simulink model "winter_simulink"  (R2022a)
settings: Solver=FixedStepAuto  StartTime=0  StopTime=simulation.stop_time  FixedStep=simulation.time_step  RelTol=1e-3
values from neighbouring files (symbols this model uses):
  I_eq = param{1}    [main_IMM.m]    (also in parameters_old.m = rotor.I + generator.I/gearbox.ratio^2)
  lambda_vector = linspace(lambda_range(1), lambda_range(2), lambda_item)    [parameters_old.m]
  omega_rated = rated_values(2)    [parameters_old.m]
  pitch_range = deg2rad([-15 90])    [parameters_old.m]
  pitch_vector = linspace(pitch_range(1), pitch_range(2), pitch_item)    [parameters_old.m]
  rho = param{2}    [main_IMM.m]    (also in parameters_old.m = 1.225)
undefined symbols (not defined in the file or in its folder): blade, Gc, gearbox, generator, lookup_cP, omega_r, Riq, rotor, wind, Yiq
settings Model: Creator=Niccolò  LastModifiedBy=Niccolò

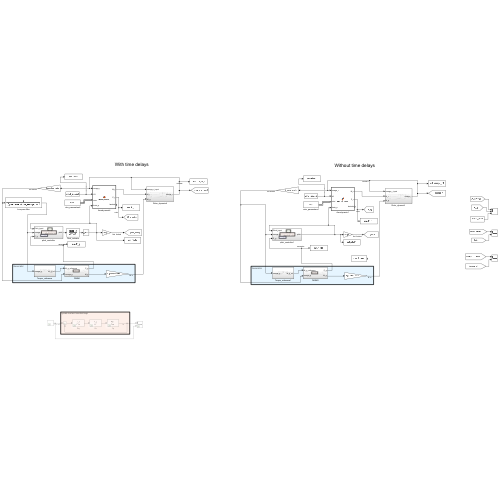
[thumbnail: Simulink's stored preview of the top-level diagram]
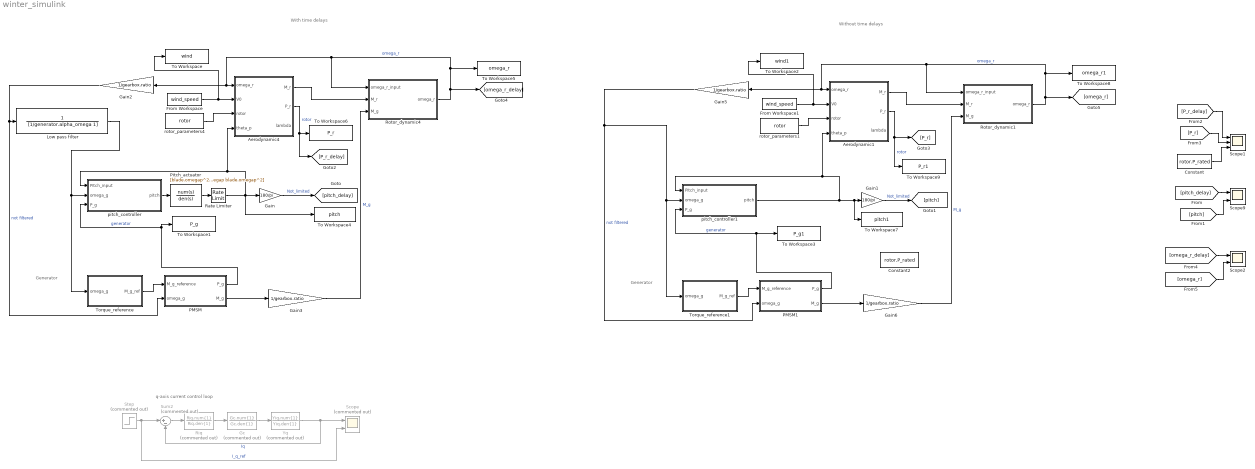
== system winter_simulink ==
  note: Generator
  note: With time delays
  note: q-axis current control loop
  note: Generator
  note: Without time delays
  Aerodynamic1 : MATLAB Function  TreatAsAtomicUnit=on
  Aerodynamic4 : MATLAB Function  TreatAsAtomicUnit=on
  Constant : Constant  Value=rotor.P_rated
  Constant2 : Constant  Value=rotor.P_rated
  From Workspace : FromWorkspace  VariableName=wind_speed  SampleTime=1/wind.sample_f
  From Workspace1 : FromWorkspace  VariableName=wind_speed  SampleTime=1/wind.sample_f
  Gain : Gain  Gain=180/pi
  Gain1 : Gain  Gain=180/pi
  Gain{2..3,5..6} (4 alike) : Gain  Gain=1/gearbox.ratio
  Gc : TransferFcn  Commented=on  Numerator=Gc.num{1}  Denominator=Gc.den{1}
  Low pass filter : TransferFcn  Denominator=[1/generator.alpha_omega 1]
  PMSM : Subsystem
  PMSM1 : Subsystem
  Pitch_actuator : TransferFcn  Numerator=[blade.omegap^2]  Denominator=[1 2*blade.zetap*blade.omegap blade.omegap^2]
  Rate Limiter : RateLimiter  RisingSlewLimit=blade.pitch_rate  FallingSlewLimit=-blade.pitch_rate  SampleTimeMode=inherited
  Riq : TransferFcn  Commented=on  Numerator=Riq.num{1}  Denominator=Riq.den{1}
  Rotor_dynamic1 : Subsystem
  Rotor_dynamic4 : Subsystem
  Scope : Scope  Commented=on  NumInputPorts=2
  Scope1 : Scope  NumInputPorts=3
  Scope2 : Scope  NumInputPorts=2
  Scope9 : Scope  NumInputPorts=2
  Step : Step  Commented=on  SampleTime=0
  Sum2 : Sum  Commented=on  Inputs=|+-
  To Workspace : ToWorkspace  VariableName=wind  SaveFormat=Timeseries  SampleTime=-1
  To Workspace1 : ToWorkspace  VariableName=P_g  SaveFormat=Timeseries  SampleTime=-1
  To Workspace2 : ToWorkspace  VariableName=wind1  SaveFormat=Timeseries  SampleTime=-1
  To Workspace3 : ToWorkspace  VariableName=P_g1  SaveFormat=Timeseries  SampleTime=-1
  To Workspace4 : ToWorkspace  VariableName=pitch  SaveFormat=Timeseries  SampleTime=-1
  To Workspace5 : ToWorkspace  VariableName=omega_r  SaveFormat=Timeseries  SampleTime=-1
  To Workspace6 : ToWorkspace  VariableName=P_r  SaveFormat=Timeseries  SampleTime=-1
  To Workspace7 : ToWorkspace  VariableName=pitch1  SaveFormat=Timeseries  SampleTime=-1
  To Workspace8 : ToWorkspace  VariableName=omega_r1  SaveFormat=Timeseries  SampleTime=-1
  To Workspace9 : ToWorkspace  VariableName=P_r1  SaveFormat=Timeseries  SampleTime=-1
  Torque_reference : Subsystem
  Torque_reference1 : Subsystem
  Yq : TransferFcn  Commented=on  Numerator=Yiq.num{1}  Denominator=Yiq.den{1}
  pitch_controller : Subsystem
  pitch_controller1 : Subsystem
  rotor_parameters1 : Constant  Value=rotor  OutDataTypeStr=Bus: rotor_bus
  rotor_parameters4 : Constant  Value=rotor  OutDataTypeStr=Bus: rotor_bus
  wires:
  Aerodynamic4/1(M_r) -> Rotor_dynamic4/2(M_r)
  From Workspace/1 -> To Workspace/1, Aerodynamic4/2(V0)
  rotor_parameters4/1 -> Aerodynamic4/3(rotor)
  Gain2/1 -> PMSM/2(omega_g), Low pass filter/1  "not filtered"
  Rotor_dynamic4/1(omega_r) -> [omega_r_delay], Rotor_dynamic4/1(omega_r_input), Gain2/1, Aerodynamic4/1(omega_r), To Workspace5/1  "omega_r"
  Aerodynamic4/2(P_r) -> [P_r_delay], To Workspace6/1  "rotor"
  Gain/1 -> [pitch_delay]  "Not_limited"
  PMSM/1(P_g) -> To Workspace1/1, pitch_controller/3(P_g)  "generator"
  Torque_reference/1(M_g_ref) -> PMSM/1(M_g_reference)
  pitch_controller/1(pitch) -> Pitch_actuator/1
  PMSM/2(M_g) -> Gain3/1
  Gain3/1 -> Rotor_dynamic4/3(M_g)  "M_g"
  Step/1 -> Scope/2, Sum2/1  "I_q_ref"
  Gc/1 -> Yq/1
  Riq/1 -> Gc/1
  Yq/1 -> Scope/1, Sum2/2  "Iq"
  Sum2/1 -> Riq/1
  Low pass filter/1 -> Torque_reference/1(omega_g), pitch_controller/2(omega_g)
  Pitch_actuator/1 -> Rate Limiter/1
  Rate Limiter/1 -> Aerodynamic4/4(theta_p), pitch_controller/1(Pitch_input), Gain/1, To Workspace4/1
  pitch_controller1/1(pitch) -> To Workspace7/1, Gain1/1, Aerodynamic1/4(theta_p), pitch_controller1/1(Pitch_input)
  PMSM1/2(M_g) -> Gain6/1
  PMSM1/1(P_g) -> pitch_controller1/3(P_g), To Workspace3/1  "generator"
  Gain6/1 -> Rotor_dynamic1/3(M_g)  "M_g"
  Torque_reference1/1(M_g_ref) -> PMSM1/1(M_g_reference)
  rotor_parameters1/1 -> Aerodynamic1/3(rotor)
  Gain1/1 -> [pitch]  "Not_limited"
  Gain5/1 -> Torque_reference1/1(omega_g), pitch_controller1/2(omega_g), PMSM1/2(omega_g)  "not filtered"
  Aerodynamic1/2(P_r) -> [P_r], To Workspace9/1  "rotor"
  Rotor_dynamic1/1(omega_r) -> [omega_r], Rotor_dynamic1/1(omega_r_input), Gain5/1, Aerodynamic1/1(omega_r), To Workspace8/1  "omega_r"
  From Workspace1/1 -> To Workspace2/1, Aerodynamic1/2(V0)
  Aerodynamic1/1(M_r) -> Rotor_dynamic1/2(M_r)
  [pitch_delay] -> Scope9/1
  [pitch] -> Scope9/2
  [P_r_delay] -> Scope1/1
  [P_r] -> Scope1/2
  Constant/1 -> Scope1/3
  [omega_r_delay] -> Scope2/1
  [omega_r] -> Scope2/2

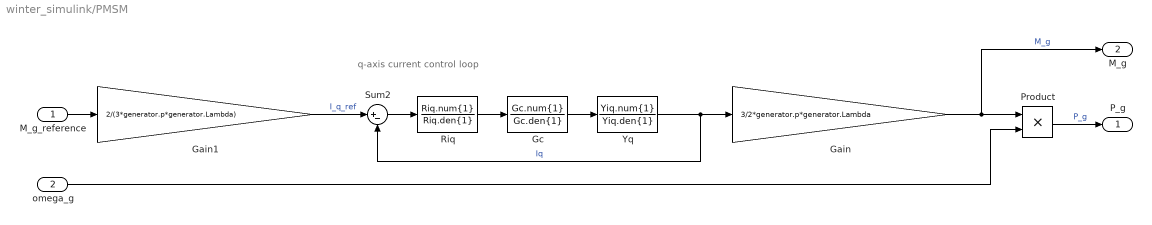
== system winter_simulink/PMSM ==
  note: q-axis current control loop
  M_g_reference : Inport
  omega_g : Inport  Port=2
  Gain : Gain  Gain=3/2*generator.p*generator.Lambda
  Gain1 : Gain  Gain=2/(3*generator.p*generator.Lambda)
  Gc : TransferFcn  Numerator=Gc.num{1}  Denominator=Gc.den{1}
  Product : Product
  Riq : TransferFcn  Numerator=Riq.num{1}  Denominator=Riq.den{1}
  Sum2 : Sum  Inputs=|+-
  Yq : TransferFcn  Numerator=Yiq.num{1}  Denominator=Yiq.den{1}
  P_g : Outport
  M_g : Outport  Port=2
  wires:
  Gc/1 -> Yq/1
  M_g_reference/1 -> Gain1/1
  Gain/1 -> M_g/1, Product/1  "M_g"
  Riq/1 -> Gc/1
  Sum2/1 -> Riq/1
  Yq/1 -> Gain/1, Sum2/2  "Iq"
  Product/1 -> P_g/1  "P_g"
  omega_g/1 -> Product/2
  Gain1/1 -> Sum2/1  "I_q_ref"

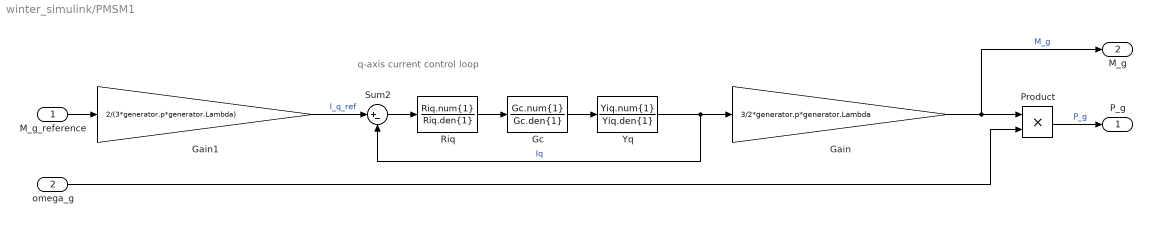
== system winter_simulink/PMSM1 ==
  note: q-axis current control loop
  M_g_reference : Inport
  omega_g : Inport  Port=2
  Gain : Gain  Gain=3/2*generator.p*generator.Lambda
  Gain1 : Gain  Gain=2/(3*generator.p*generator.Lambda)
  Gc : TransferFcn  Numerator=Gc.num{1}  Denominator=Gc.den{1}
  Product : Product
  Riq : TransferFcn  Numerator=Riq.num{1}  Denominator=Riq.den{1}
  Sum2 : Sum  Inputs=|+-
  Yq : TransferFcn  Numerator=Yiq.num{1}  Denominator=Yiq.den{1}
  P_g : Outport
  M_g : Outport  Port=2
  wires:
  Gc/1 -> Yq/1
  M_g_reference/1 -> Gain1/1
  Gain/1 -> M_g/1, Product/1  "M_g"
  Riq/1 -> Gc/1
  Sum2/1 -> Riq/1
  Yq/1 -> Gain/1, Sum2/2  "Iq"
  Product/1 -> P_g/1  "P_g"
  omega_g/1 -> Product/2
  Gain1/1 -> Sum2/1  "I_q_ref"

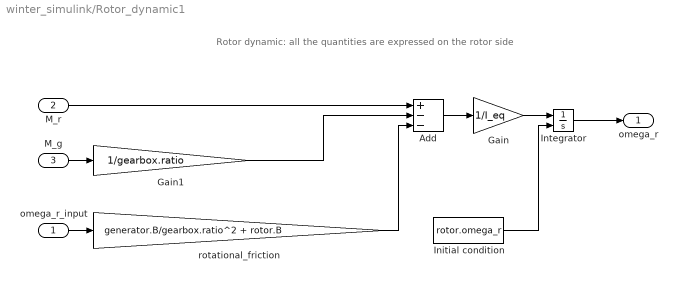
== system winter_simulink/Rotor_dynamic1 ==
  note: Rotor dynamic: all the quantities are expressed on the rotor side
  omega_r_input : Inport
  M_r : Inport  Port=2
  M_g : Inport  Port=3
  Add : Sum  Inputs=+--
  Gain : Gain  Gain=1/I_eq
  Gain1 : Gain  Gain=1/gearbox.ratio
  Initial condition : Constant  Value=rotor.omega_r
  Integrator : Integrator  InitialConditionSource=external  InitialCondition=omega_r
  rotational_friction : Gain  Gain=generator.B/gearbox.ratio^2 + rotor.B
  omega_r : Outport
  wires:
  Add/1 -> Gain/1
  Gain/1 -> Integrator/1
  M_r/1 -> Add/1
  Initial condition/1 -> Integrator/2
  omega_r_input/1 -> rotational_friction/1
  rotational_friction/1 -> Add/3
  M_g/1 -> Gain1/1
  Gain1/1 -> Add/2
  Integrator/1 -> omega_r/1

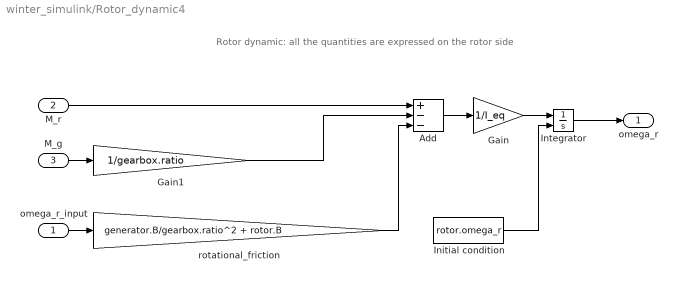
== system winter_simulink/Rotor_dynamic4 ==
  note: Rotor dynamic: all the quantities are expressed on the rotor side
  omega_r_input : Inport
  M_r : Inport  Port=2
  M_g : Inport  Port=3
  Add : Sum  Inputs=+--
  Gain : Gain  Gain=1/I_eq
  Gain1 : Gain  Gain=1/gearbox.ratio
  Initial condition : Constant  Value=rotor.omega_r
  Integrator : Integrator  InitialConditionSource=external  InitialCondition=omega_r
  rotational_friction : Gain  Gain=generator.B/gearbox.ratio^2 + rotor.B
  omega_r : Outport
  wires:
  Add/1 -> Gain/1
  Gain/1 -> Integrator/1
  M_r/1 -> Add/1
  Initial condition/1 -> Integrator/2
  omega_r_input/1 -> rotational_friction/1
  rotational_friction/1 -> Add/3
  M_g/1 -> Gain1/1
  Gain1/1 -> Add/2
  Integrator/1 -> omega_r/1

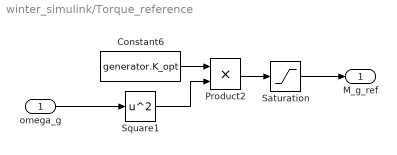
== system winter_simulink/Torque_reference ==
  omega_g : Inport
  Constant6 : Constant  Value=generator.K_opt
  Product2 : Product
  Saturation : Saturate  UpperLimit=rotor.P_rated*gearbox.ratio/omega_rated  LowerLimit=0
  Square1 : Math  Operator=square
  M_g_ref : Outport
  wires:
  Product2/1 -> Saturation/1
  omega_g/1 -> Square1/1
  Square1/1 -> Product2/2
  Constant6/1 -> Product2/1
  Saturation/1 -> M_g_ref/1

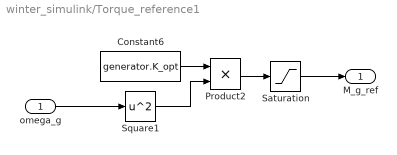
== system winter_simulink/Torque_reference1 ==
  omega_g : Inport
  Constant6 : Constant  Value=generator.K_opt
  Product2 : Product
  Saturation : Saturate  UpperLimit=rotor.P_rated*gearbox.ratio/omega_rated  LowerLimit=0
  Square1 : Math  Operator=square
  M_g_ref : Outport
  wires:
  Product2/1 -> Saturation/1
  omega_g/1 -> Square1/1
  Square1/1 -> Product2/2
  Constant6/1 -> Product2/1
  Saturation/1 -> M_g_ref/1

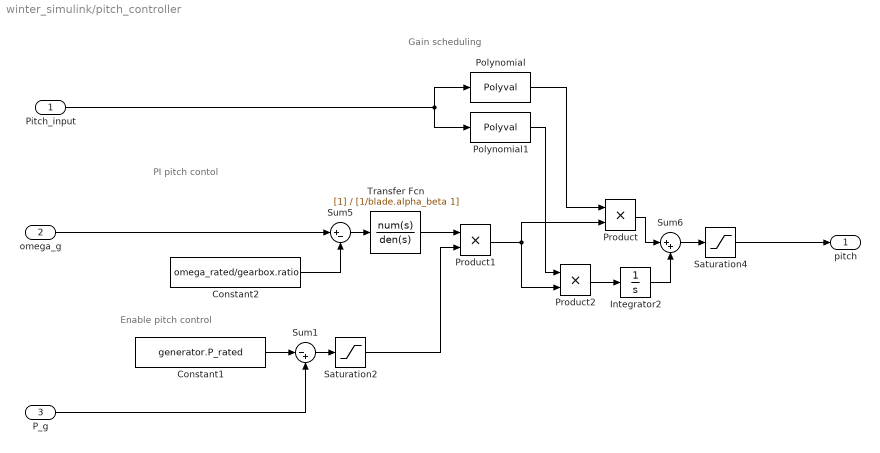
== system winter_simulink/pitch_controller ==
  note: Gain scheduling
  note: Enable pitch control
  note: PI pitch contol
  Pitch_input : Inport
  omega_g : Inport  Port=2
  P_g : Inport  Port=3
  Constant1 : Constant  Value=generator.P_rated
  Constant2 : Constant  Value=omega_rated/gearbox.ratio
  Integrator2 : Integrator
  Polynomial : Polyval  Coefs=blade.kp_schedule
  Polynomial1 : Polyval  Coefs=blade.ki_schedule
  Product : Product
  Product1 : Product
  Product2 : Product
  Saturation2 : Saturate  UpperLimit=1  LowerLimit=0
  Saturation4 : Saturate  UpperLimit=pitch_range(2)  LowerLimit=pitch_range(1)
  Sum1 : Sum  Inputs=|-+
  Sum5 : Sum  Inputs=|+-
  Sum6 : Sum  Inputs=|++
  Transfer Fcn : TransferFcn  Denominator=[1/blade.alpha_beta 1]
  pitch : Outport
  wires:
  Saturation4/1 -> pitch/1
  omega_g/1 -> Sum5/1
  Sum1/1 -> Saturation2/1
  P_g/1 -> Sum1/2
  Sum6/1 -> Saturation4/1
  Product/1 -> Sum6/1
  Product2/1 -> Integrator2/1
  Product1/1 -> Product2/2, Product/2
  Constant2/1 -> Sum5/2
  Constant1/1 -> Sum1/1
  Saturation2/1 -> Product1/2
  Sum5/1 -> Transfer Fcn/1
  Polynomial/1 -> Product/1
  Pitch_input/1 -> Polynomial/1, Polynomial1/1
  Integrator2/1 -> Sum6/2
  Transfer Fcn/1 -> Product1/1
  Polynomial1/1 -> Product2/1

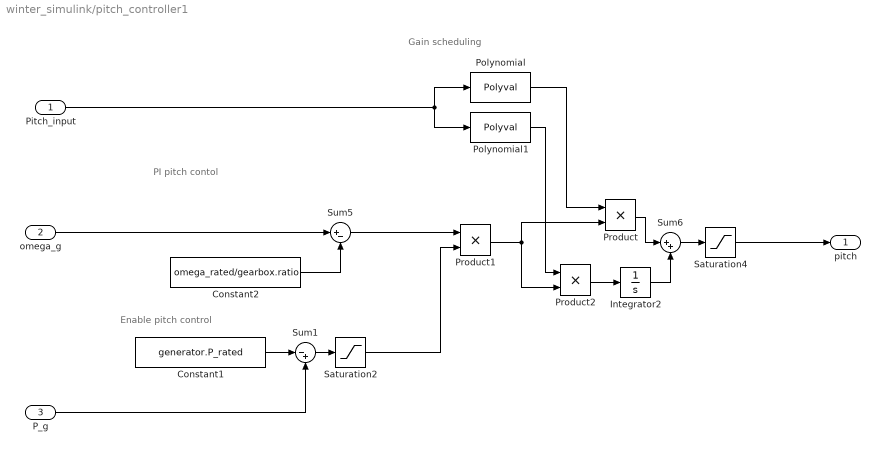
== system winter_simulink/pitch_controller1 ==
  note: Gain scheduling
  note: Enable pitch control
  note: PI pitch contol
  Pitch_input : Inport
  omega_g : Inport  Port=2
  P_g : Inport  Port=3
  Constant1 : Constant  Value=generator.P_rated
  Constant2 : Constant  Value=omega_rated/gearbox.ratio
  Integrator2 : Integrator
  Polynomial : Polyval  Coefs=blade.kp_schedule
  Polynomial1 : Polyval  Coefs=blade.ki_schedule
  Product : Product
  Product1 : Product
  Product2 : Product
  Saturation2 : Saturate  UpperLimit=1  LowerLimit=0
  Saturation4 : Saturate  UpperLimit=pitch_range(2)  LowerLimit=pitch_range(1)
  Sum1 : Sum  Inputs=|-+
  Sum5 : Sum  Inputs=|+-
  Sum6 : Sum  Inputs=|++
  pitch : Outport
  wires:
  Saturation4/1 -> pitch/1
  omega_g/1 -> Sum5/1
  Sum1/1 -> Saturation2/1
  P_g/1 -> Sum1/2
  Sum6/1 -> Saturation4/1
  Product/1 -> Sum6/1
  Product2/1 -> Integrator2/1
  Product1/1 -> Product2/2, Product/2
  Constant2/1 -> Sum5/2
  Constant1/1 -> Sum1/1
  Saturation2/1 -> Product1/2
  Polynomial/1 -> Product/1
  Pitch_input/1 -> Polynomial/1, Polynomial1/1
  Integrator2/1 -> Sum6/2
  Sum5/1 -> Product1/1
  Polynomial1/1 -> Product2/1

== matlab function winter_simulink/Aerodynamic4 ==
  data: omega_r input; V0 input; M_r output; P_r output; rho parameter; rotor input; theta_p input; lambda_vector parameter; pitch_vector parameter; lookup_cP parameter; lambda output
function [M_r, P_r, lambda] = Aerodynamic(omega_r, V0, rho, rotor, ...
  theta_p, lambda_vector, pitch_vector, lookup_cP) 

R = rotor.R;                  % rotor radius [m]

% retrive the cP from the look-up table
lambda = omega_r*R/V0;                                                
cP = interp2(lambda_vector, pitch_vector, lookup_cP, lambda, theta_p);

P_r = 0.5*rho*V0^3*pi*R^2*cP; % rotor power [W]
M_r = P_r/omega_r;            % rotor torque [Nm]

== matlab function winter_simulink/Aerodynamic1 ==
  data: omega_r input; V0 input; M_r output; P_r output; rho parameter; rotor input; theta_p input; lambda_vector parameter; pitch_vector parameter; lookup_cP parameter; lambda output
function [M_r, P_r, lambda] = Aerodynamic(omega_r, V0, rho, rotor, ...
  theta_p, lambda_vector, pitch_vector, lookup_cP) 

R = rotor.R;                  % rotor radius [m]

% retrive the cP from the look-up table
lambda = omega_r*R/V0;                                                
cP = interp2(lambda_vector, pitch_vector, lookup_cP, lambda, theta_p);

P_r = 0.5*rho*V0^3*pi*R^2*cP; % rotor power [W]
M_r = P_r/omega_r;            % rotor torque [Nm]
